simulink model "dq0_using_fcn"  (R2025a)
settings: Solver=VariableStepAuto  StartTime=0.0  StopTime=0.1  MaxStep=1e-6  RelTol=1e-3
libraries: spspowerguiLib x1
settings Model: Creator=prajw  LastModifiedBy=prajw

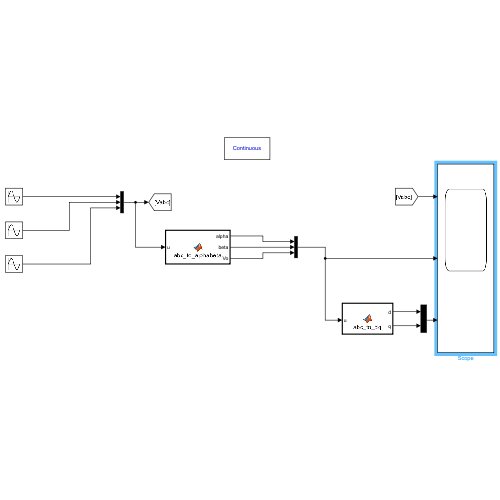
[thumbnail: Simulink's stored preview of the top-level diagram]
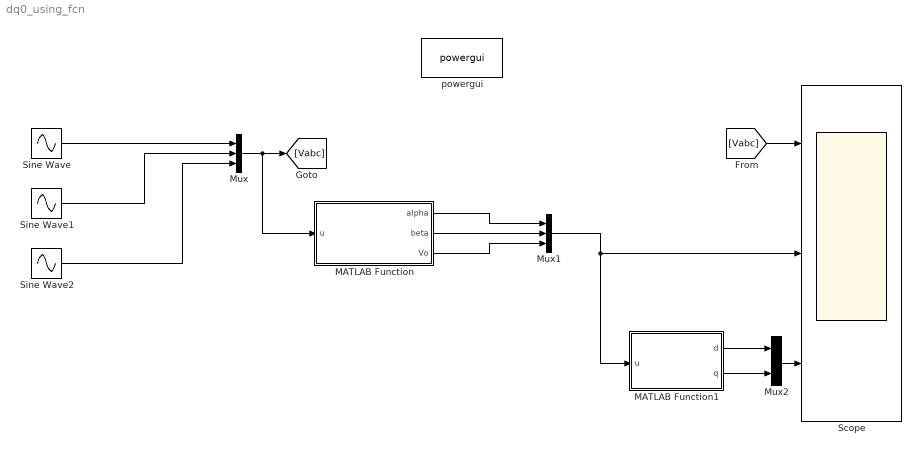
== system dq0_using_fcn ==
  MATLAB Function : MATLAB Function  TreatAsAtomicUnit=on
  MATLAB Function1 : MATLAB Function  TreatAsAtomicUnit=on
  Mux : Mux  Inputs=3
  Mux1 : Mux  Inputs=3
  Mux2 : Mux  Inputs=2
  Scope : Scope  NumInputPorts=3
      settings: ActiveDisplayString=3  ActiveDisplayYMinimum=-404.35907634570759  ActiveDisplayYMaximum=404.35907634570754  YLabel=Vdq
  Sine Wave : Sin  Amplitude=230*sqrt(2)  Frequency=2*pi*50  SampleTime=0
  Sine Wave1 : Sin  Amplitude=230*sqrt(2)  Frequency=2*pi*50  Phase=2*pi/3  SampleTime=0
  Sine Wave2 : Sin  Amplitude=230*sqrt(2)  Frequency=2*pi*50  Phase=-2*pi/3  SampleTime=0
  powergui : spspowerguiLib/powergui  Priority=1  SimulationMode=Continuous  SampleTime=50e-6  frequency=60  Iterations=50  frequencyindice=60  Pbase=100e6  ErrMax=1e-4  UnitsV=kV  UnitsW=MW  buscounter=0  FunctionMessages=off  echomessages=off  EnableUseOfTLC=off  CurrentSourceSwitches=off  DisableSnubberDevices=off  DisableRonSwitches=off  DisableVfSwitches=off  DisplayEquations=off  AutomaticDiscreteSolvers=off  SolverType=Tustin/Backward Euler (TBE)  Interpol=off  ExternalGateDelay=off  methode=off  Ts=100  x0status=blocks  SPID=on  SwTol=0  HookPort=off  NonlinearTolerance=1e-4  nMaxIteration=100  ContinueOnMaxIteration=off  RestoreLinks=warning  ResistiveCurrentMeasurement=off  Frange=[0:2:500]  Ylog=off  Xlog=on  ShowGrid=off  save=off  variable=ZData  structure=0  ZoomFFT=off  StartTime=0.0  cycles=1  DisplayStyle=1  fundamental=60  FreqAxis=off  MaxFrequency=1000  frequencyindicesteady=1  RmsSteady=1  display=off
  wires:
  Sine Wave/1 -> Mux/1
  Sine Wave1/1 -> Mux/2
  Sine Wave2/1 -> Mux/3
  [Vabc] -> Scope/1
  Mux/1 -> [Vabc], MATLAB Function/1(u)
  MATLAB Function/1(alpha) -> Mux1/1
  MATLAB Function/2(beta) -> Mux1/2
  MATLAB Function/3(Vo) -> Mux1/3
  Mux1/1 -> MATLAB Function1/1(u), Scope/2
  MATLAB Function1/1(d) -> Mux2/1
  MATLAB Function1/2(q) -> Mux2/2
  Mux2/1 -> Scope/3

== matlab function dq0_using_fcn/MATLAB Function ==
  data: u input; alpha output; beta output; Vo output
function [alpha, beta, Vo] = abc_to_alphabeta(u)
% Clarke Transformation (ABC → αβ)

Va = u(1);
Vb = u(2);
Vc = u(3);

alpha = (2/3)*(Va - 0.5*Vb - 0.5*Vc);
beta  = (2/3)*( (sqrt(3)/2)*(Vb - Vc) );
Vo= (2/3)*(1/2)*(Va + Vb + Vc)
end

== matlab function dq0_using_fcn/MATLAB Function1 ==
  data: u input; d output; q output
function [d, q] = abc_to_dq(u)
alpha=u(1);
beta= u(2);
%% Angle from αβ
theta = atan2(beta, alpha);   % radians, [-pi, pi]

%% Park Transform (αβ → dq)
c = cos(theta);
s = sin(theta);

d =  alpha*c + beta*s;
q = -alpha*s + beta*c;

end
